simulink model "capacitor_de_partida"  (R2024b)
settings: Solver=VariableStepAuto  StartTime=0.0  StopTime=3  RelTol=1e-3
undefined symbols (not defined in the file): Capacitor, Start
libraries: spsACVoltageSourceLib x1, spsSinglePhaseAsynchronousMachineLib x1, spsCurrentMeasurementLib x1, spspowerguiLib x1
settings Model: NumberOfSteps=10  Creator=root

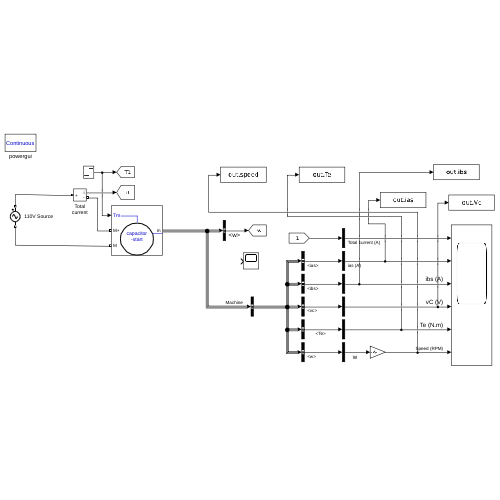
[thumbnail: Simulink's stored preview of the top-level diagram]
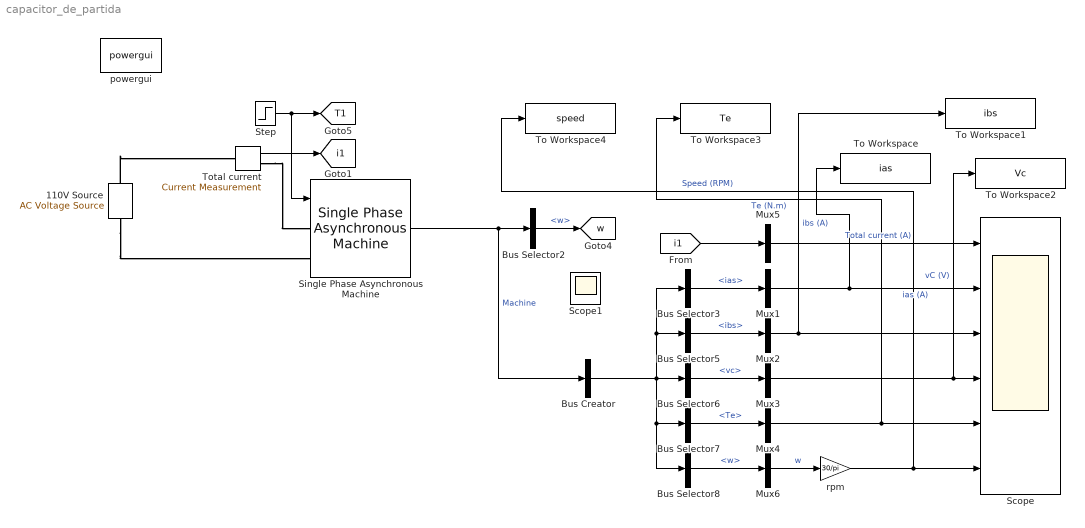
== system capacitor_de_partida ==
  110V Source : spsACVoltageSourceLib/AC Voltage Source  Amplitude=110*sqrt(2)  Phase=90  Frequency=60  SampleTime=0  Measurements=Voltage  BusType=swing  Pref=10e3  Qref=0  Qmin=-inf  Qmax=+inf
  Bus Creator : BusCreator  Inputs=1
  Bus Selector2 : BusSelector  OutputSignals=w
  Bus Selector3 : BusSelector  OutputSignals=Machine.ias
  Bus Selector5 : BusSelector  OutputSignals=Machine.ibs
  Bus Selector6 : BusSelector  OutputSignals=Machine.vc
  Bus Selector7 : BusSelector  OutputSignals=Machine.Te
  Bus Selector8 : BusSelector  OutputSignals=Machine.w
  Mux{1..6} (6 alike) : Mux  Inputs=1
  Scope : Scope  NumInputPorts=6
  Scope1 : Scope
  Single Phase Asynchronous Machine : spsSinglePhaseAsynchronousMachineLib/Single Phase Asynchronous Machine  MechanicalLoad=Torque Tm  UNITS=SI  MachineType=Capacitor-Start  MeasurementBus=on  NominalParameters="[ .25*746  110  60]"  MainWindingStator="[2.02  7.4e-3]"  MainWindingRotor="[4.12  5.6e-3]"  MutualInductance=0.177  AuxiliaryWinding=[7.14 8.54e-3]  Mechanical=[0.0146 0 2 1.18]  CapacitorStart="[2.15  255e-6]"  CapacitorRun=[0.04624 1592]  DisconnectionSpeed=75  InitialSpeed=0  DataType=SI  TsPowergui=0  TsBlock=-1
  Step : Step  Time=2  SampleTime=0
  To Workspace : ToWorkspace  VariableName=ias  SaveFormat=Timeseries  SampleTime=-1
  To Workspace1 : ToWorkspace  VariableName=ibs  SaveFormat=Timeseries  SampleTime=-1
  To Workspace2 : ToWorkspace  VariableName=Vc  SaveFormat=Timeseries  SampleTime=-1
  To Workspace3 : ToWorkspace  VariableName=Te  SaveFormat=Timeseries  SampleTime=-1
  To Workspace4 : ToWorkspace  VariableName=speed  SaveFormat=Timeseries  SampleTime=-1
  Total current : spsCurrentMeasurementLib/Current Measurement  PhasorSimulation=off  OutputType=Complex  PSBequivalent=0
  powergui : spspowerguiLib/powergui  SimulationMode=Continuous  SampleTime=1e-5  frequency=60  Iterations=50  frequencyindice=60  Pbase=100e6  ErrMax=1e-4  UnitsV=kV  UnitsW=MW  buscounter=0  FunctionMessages=off  echomessages=off  EnableUseOfTLC=off  CurrentSourceSwitches=off  DisableSnubberDevices=off  DisableRonSwitches=off  DisableVfSwitches=off  DisplayEquations=off  AutomaticDiscreteSolvers=off  SolverType=Tustin  Interpol=off  ExternalGateDelay=off  methode=off  Ts=0  x0status=blocks  SPID=on  SwTol=0  HookPort=off  NonlinearTolerance=1e-4  nMaxIteration=100  ContinueOnMaxIteration=off  RestoreLinks=warning  ResistiveCurrentMeasurement=off  Frange=[0:2:500]  Ylog=off  Xlog=on  ShowGrid=off  save=off  variable=ZData  structure=0  ZoomFFT=on  StartTime=0.0  cycles=1  DisplayStyle=1  fundamental=60  FreqAxis=off  MaxFrequency=1000  frequencyindicesteady=1  RmsSteady=1  display=off
  rpm : Gain  Gain=30/pi  SaturateOnIntegerOverflow=on  OutDataTypeStr=Inherit: Same as input  ParamDataTypeStr=Inherit: Same as input
  tag scope: T1=global, i1=global, w=global
  wires:
  Total current/1 -> [i1]
  Bus Selector3/1 -> Mux1/1  "<ias>"
  rpm/1 -> To Workspace4/1, Scope/6  "Speed (RPM)"
  Bus Selector7/1 -> Mux4/1  "<Te>"
  Bus Selector6/1 -> Mux3/1  "<vc>"
  Bus Selector8/1 -> Mux6/1  "<w>"
  Bus Selector5/1 -> Mux2/1  "<ibs>"
  Bus Creator/1 -> Bus Selector8/1, Bus Selector7/1, Bus Selector6/1, Bus Selector5/1, Bus Selector3/1
  Mux6/1 -> rpm/1  "w"
  Single Phase Asynchronous Machine/1 -> Bus Selector2/1, Bus Creator/1  "Machine"
  Bus Selector2/1 -> [w]  "<w>"
  Mux2/1 -> Scope/3, To Workspace1/1  "ibs (A)"
  Mux4/1 -> To Workspace3/1, Scope/5  "Te (N.m)"
  Mux3/1 -> To Workspace2/1, Scope/4  "vC (V)"
  [i1] -> Mux5/1
  Step/1 -> Single Phase Asynchronous Machine/1, [T1]
  Mux5/1 -> Scope/1  "Total current (A)"
  Mux1/1 -> To Workspace/1, Scope/2  "ias (A)"
  connections:
  Total current/RConn1 -- Single Phase Asynchronous Machine/LConn1
  110V Source/RConn1 -- Total current/LConn1
  110V Source/LConn1 -- Single Phase Asynchronous Machine/LConn2
